simulink subsystem "tehrani_tissue_mass_balance_v3"  (R2020b)
settings: Solver=VariableStepAuto  StartTime=0.0  StopTime=10.0  RelTol=1e-3
settings Model: Creator=RH  LastModifiedBy=fonck

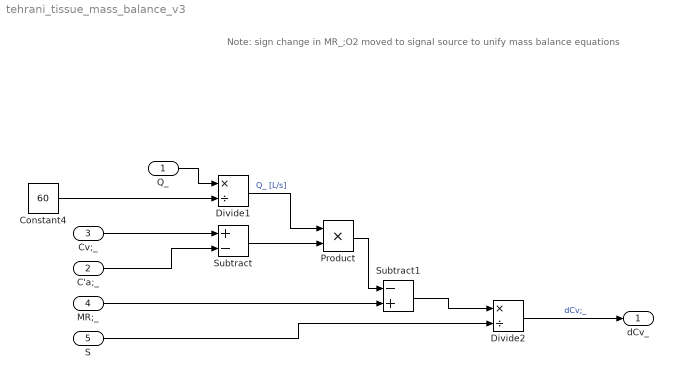
== system tehrani_tissue_mass_balance_v3 ==
  note: Note: sign change in MR_;O2 moved to signal source to unify mass balance equations
  Q_ : Inport  Unit=L/min
  C'a;_ : Inport  Port=2  Unit=1
  Cv;_ : Inport  Port=3  Unit=1
  MR;_ : Inport  Port=4  Unit=L/s
  S : Inport  Port=5  Unit=L
  Constant4 : Constant  Value=60
  Divide1 : Product  Inputs=*/
  Divide2 : Product  Inputs=*/
  Product : Product
  Subtract : Sum  Inputs=+-
  Subtract1 : Sum  Inputs=-+
  dCv_ : Outport  Unit=1/s
  wires:
  Divide2/1 -> dCv_/1  "dCv;_"
  Product/1 -> Subtract1/1
  Constant4/1 -> Divide1/2
  Cv;_/1 -> Subtract/1
  Subtract1/1 -> Divide2/1
  Subtract/1 -> Product/2
  C'a;_/1 -> Subtract/2
  Q_/1 -> Divide1/1
  Divide1/1 -> Product/1  "Q_ [L/s]"
  MR;_/1 -> Subtract1/2
  S/1 -> Divide2/2
